simulink model "odeSimulink_Demo"  (R2017b)
settings: Solver=VariableStepAuto  StartTime=0.0  StopTime=10.0  RelTol=1e-3
settings Model: Creator=javed  LastModifiedBy=javed

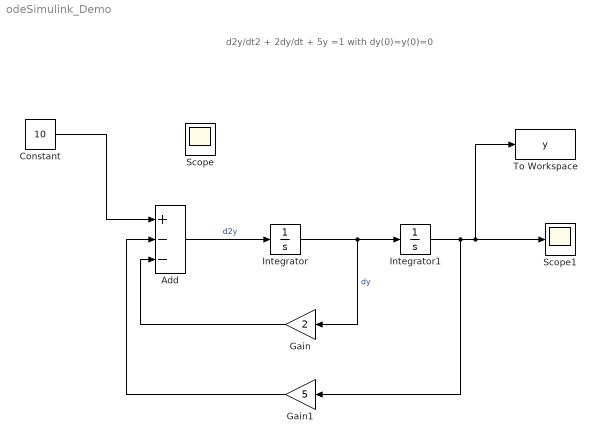
== system odeSimulink_Demo ==
  note: d2y/dt2 + 2dy/dt + 5y =1
      |
      | with dy(0)=y(0)=0
  Add : Sum  Inputs=+--
  Constant : Constant  Value=10
  Gain : Gain  Gain=2
  Gain1 : Gain  Gain=5
  Integrator : Integrator
  Integrator1 : Integrator
  Scope1 : Scope
  To Workspace : ToWorkspace  VariableName=y  SampleTime=-1
  Scope : Scope
  wires:
  Integrator/1 -> Gain/1, Integrator1/1  "dy"
  Constant/1 -> Add/1
  Add/1 -> Integrator/1  "d2y"
  Integrator1/1 -> Gain1/1, To Workspace/1, Scope1/1
  Gain/1 -> Add/3
  Gain1/1 -> Add/2
